simulink model "PWMSimulink"  (R2023b)
settings: Solver=ode23s  StartTime=0.0  StopTime=0.01  RelTol=1e-3
values from neighbouring files (symbols this model uses):
  C = 10e-6    (= 1e-05)    [PWM.m]
  d = 0.4    [PWM.m]
  L = 0.002    [PWM.m]
  R = 10    [PWM.m]

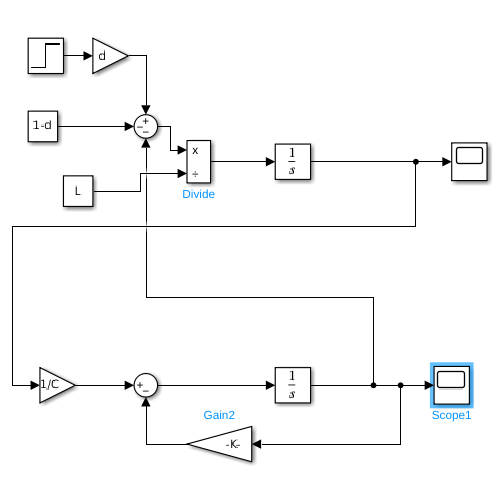
[thumbnail: Simulink's stored preview of the top-level diagram]
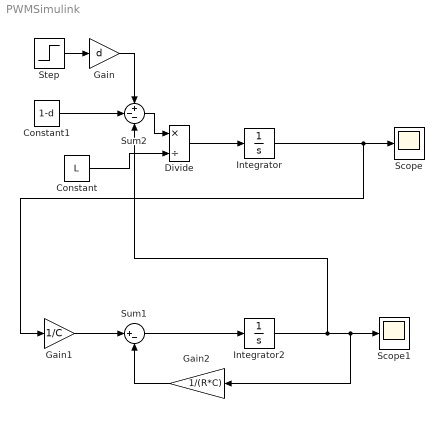
== system PWMSimulink ==
  Constant : Constant  Value=L
  Constant1 : Constant  Value=1-d
  Divide : Product  Inputs=*/
  Gain : Gain  Gain=d
  Gain1 : Gain  Gain=1/C
  Gain2 : Gain  Gain=1/(R*C)
  Integrator : Integrator
  Integrator2 : Integrator
  Scope : Scope
  Scope1 : Scope
  Step : Step  Time=0  After=32  SampleTime=0
  Sum1 : Sum  Inputs=|+-
  Sum2 : Sum  Inputs=+--
  wires:
  Integrator/1 -> Gain1/1, Scope/1
  Integrator2/1 -> Gain2/1, Scope1/1, Sum2/3
  Sum1/1 -> Integrator2/1
  Gain2/1 -> Sum1/2
  Gain1/1 -> Sum1/1
  Divide/1 -> Integrator/1
  Sum2/1 -> Divide/1
  Constant/1 -> Divide/2
  Constant1/1 -> Sum2/2
  Step/1 -> Gain/1
  Gain/1 -> Sum2/1
